simulink model "lead-lag"  (R2022b)
settings: Solver=VariableStepAuto  StartTime=0.0  StopTime=10.0  RelTol=1e-3
libraries: simulink x2
settings Model: Creator=mluser  LastModifiedBy=mluser

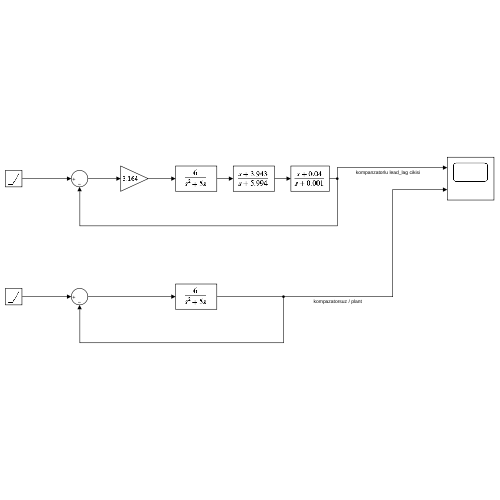
[thumbnail: Simulink's stored preview of the top-level diagram]
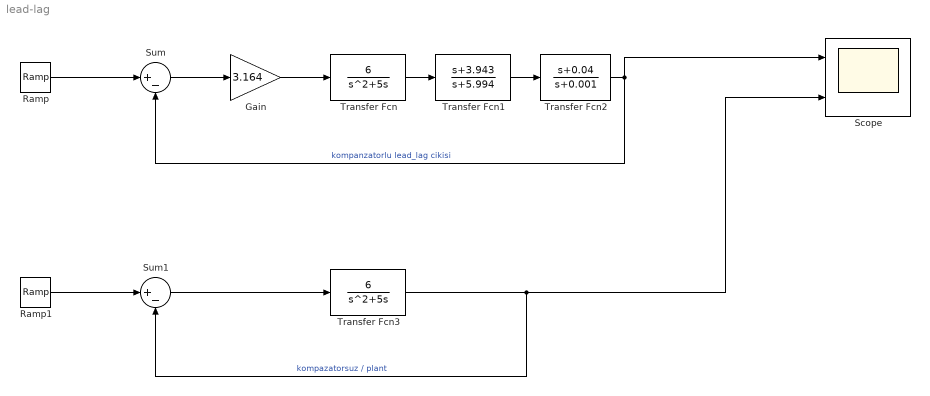
== system lead-lag ==
  Gain : Gain  Gain=3.164
  Ramp : simulink/Sources/Ramp  slope=1  start=0  InitialOutput=0
  Ramp1 : simulink/Sources/Ramp  slope=1  start=0  InitialOutput=0
  Scope : Scope  NumInputPorts=2
  Sum : Sum  Inputs=|+-
  Sum1 : Sum  Inputs=|+-
  Transfer Fcn : TransferFcn  Numerator=[6]  Denominator=[1 5 0]
  Transfer Fcn1 : TransferFcn  Numerator=[1 3.943]  Denominator=[1 5.994]
  Transfer Fcn2 : TransferFcn  Numerator=[1 0.04]  Denominator=[1 0.001]
  Transfer Fcn3 : TransferFcn  Numerator=[6]  Denominator=[1 5 0]
  wires:
  Ramp/1 -> Sum/1
  Sum/1 -> Gain/1
  Gain/1 -> Transfer Fcn/1
  Transfer Fcn/1 -> Transfer Fcn1/1
  Transfer Fcn1/1 -> Transfer Fcn2/1
  Transfer Fcn2/1 -> Sum/2, Scope/1  "kompanzatorlu lead_lag cikisi"
  Ramp1/1 -> Sum1/1
  Sum1/1 -> Transfer Fcn3/1
  Transfer Fcn3/1 -> Sum1/2, Scope/2  "kompazatorsuz / plant"
